simulink model "model_2"  (R2019b)
settings: Solver=VariableStepAuto  StartTime=0.0  StopTime=time  RelTol=1e-3
values from neighbouring files (symbols this model uses):
  Cs = tf([c2 c1 c0], [1 0 0])    [params2.m]
  Gs = tf(a, [tau 1])    [params2.m]
  slope = (y2 - y1)/(x2 - x1)    (= 0.1)    [params2.m]
  time = 1000    [params2.m]    (also in plot_2.m = transpose(out.Responses.time))
  y1 = 35    [params2.m]
undefined symbols (not defined in the file or in its folder): T0
libraries: simulink x2
settings Model: Creator=adityaaaap  LastModifiedBy=adityaaaap

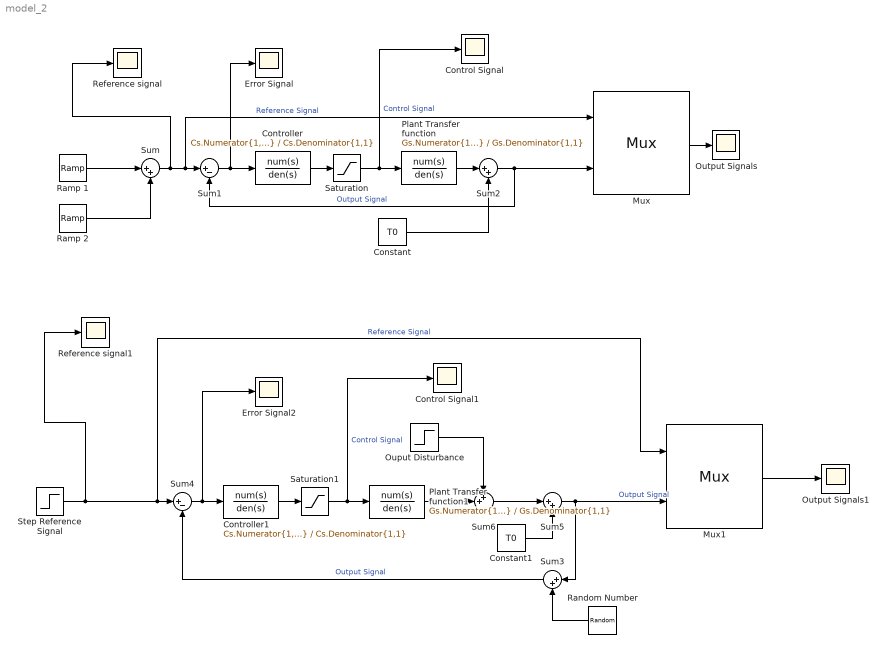
== system model_2 ==
  Constant : Constant  Value=T0
  Constant1 : Constant  Value=T0
  Control Signal : Scope
  Control Signal1 : Scope
  Controller : TransferFcn  Numerator=Cs.Numerator{1,1}  Denominator=Cs.Denominator{1,1}
  Controller1 : TransferFcn  Numerator=Cs.Numerator{1,1}  Denominator=Cs.Denominator{1,1}
  Error Signal : Scope
  Error Signal2 : Scope
  Mux : Mux  Inputs=2
      settings: DisplayOption=signals
  Mux1 : Mux  Inputs=2
      settings: DisplayOption=signals
  Ouput Disturbance : Step  Time=time/2  After=-5  SampleTime=0
  Output Signals : Scope
  Output Signals1 : Scope
  Plant Transfer function : TransferFcn  Numerator=Gs.Numerator{1,1}  Denominator=Gs.Denominator{1,1}
  Plant Transfer function1 : TransferFcn  Numerator=Gs.Numerator{1,1}  Denominator=Gs.Denominator{1,1}
  Ramp 1 : simulink/Sources/Ramp  slope=slope  start=x1  InitialOutput=0
  Ramp 2 : simulink/Sources/Ramp  slope=-slope  start=x2  InitialOutput=y1
  Random Number : RandomNumber  Variance=0.2  SampleTime=0.1
  Reference signal : Scope
  Reference signal1 : Scope
  Saturation : Saturate  UpperLimit=1  LowerLimit=0
  Saturation1 : Saturate  UpperLimit=1  LowerLimit=0
  Step Reference Signal : Step  Time=0  After=50  SampleTime=0
  Sum{,2..3,5} (4 alike) : Sum  Inputs=|++
  Sum1 : Sum  Inputs=|+-
  Sum4 : Sum  Inputs=|+-
  Sum6 : Sum  Inputs=++|
  wires:
  Ramp 1/1 -> Sum/1
  Ramp 2/1 -> Sum/2
  Sum/1 -> Reference signal/1, Mux/1, Sum1/1  "Reference Signal"
  Sum1/1 -> Error Signal/1, Controller/1
  Controller/1 -> Saturation/1
  Mux/1 -> Output Signals/1
  Plant Transfer function/1 -> Sum2/1
  Constant/1 -> Sum2/2
  Sum2/1 -> Mux/2, Sum1/2  "Output Signal"
  Saturation/1 -> Control Signal/1, Plant Transfer function/1  "Control Signal"
  Sum5/1 -> Sum3/1, Mux1/2  "Output Signal"
  Controller1/1 -> Saturation1/1
  Constant1/1 -> Sum5/2
  Step Reference Signal/1 -> Reference signal1/1, Sum4/1, Mux1/1  "Reference Signal"
  Mux1/1 -> Output Signals1/1
  Saturation1/1 -> Control Signal1/1, Plant Transfer function1/1  "Control Signal"
  Random Number/1 -> Sum3/2
  Plant Transfer function1/1 -> Sum6/2
  Sum6/1 -> Sum5/1
  Ouput Disturbance/1 -> Sum6/1
  Sum3/1 -> Sum4/2  "Output Signal"
  Sum4/1 -> Error Signal2/1, Controller1/1
